simulink model "PubIfDecisionLM_MDL"  (R2020b)
settings: configuration reference "DspaceConfig" (kept outside this file)
PostLoadFcn:
  | if any(exist('dsrtsu_mdlpostloadfcn', 'file') ~= 0), dsrtsu_mdlpostloadfcn('Execute', bdroot); end
InitFcn:
  | , if any(exist('dsmpb_private', 'file') ~= 0), dsmpb_private('dsmpb_mdlclblib', 'Init', bdroot); end,
undefined symbols (not defined in the file or in its folder): OFM_OBJ_FUSIONTYPE_E, OFM_OBJ_MOVINGSTATE_E, OFM_OBJ_ORIENTATION_E, OFM_OBJ_TYPE_E, P_LM_Cyc, P_LM_EMLHistKapRcdBufSize, P_LM_EMLHistTrajBaseDis, P_LM_EMLHistTrajPNum, P_LM_EMLKapCorrMaxThre, P_LM_EMLMinKapThre, P_LM_EMLPathDisDiffThre, P_LM_EMLQuaFiltPar, P_LM_EMLTurnActKapThre, P_LM_EMLValidQuaThre, P_LM_FntPath1Disgap, P_LM_FntPath1MinDis, P_LM_FntPath1Timegap, P_LM_FntPath2Disgap, P_LM_FntPath2MinDis, P_LM_FntPath2Timegap, P_LM_FntPath3Disgap, P_LM_FntPath3MinDis, P_LM_FntPath3Timegap, P_LM_FusBLParFiltP, P_LM_FusEVDifC2Thre, P_LM_FusEVOPath1AllVSLDisThre, P_LM_FusEVOPath1AllVSLLostNumThre, P_LM_FusEVOPath1AllVSLQuaThre, P_LM_FusEVOPath1OTLFacNLC, P_LM_FusOTLQuaThre, P_LM_FusOTLSW, P_LM_FusParC0Index, P_LM_FusParC1Index, P_LM_FusParC2Index, P_LM_FusParC3Index, P_LM_FusVSLQuaThre, P_LM_FusVSLSW, P_LM_FusVSLValidSteerWheerAngThre, P_LM_FusVSLValidVxvThre, P_LM_LaneWidth, P_LM_OTLBufTPInfoEvaFactor, P_LM_OTLObjNum, P_LM_OTLObjSelectAgeThre, P_LM_OTLObjSelectDxAssessVx, P_LM_OTLObjSelectDxThre, P_LM_OTLObjSelectVxThre, P_LM_OTLObjSelectVyAssessDx, P_LM_OTLObjSelectVyThre, P_LM_OTLTrajPntBaseDis, P_LM_OTLTrajStdThre, P_LM_VSLAvailLineNum, P_LM_VSLBLSDiffThre, P_LM_VSLBLSDisRatio, P_LM_VSLFusBLParFiltP_C1, P_LM_VSLFusBLParFiltP_C2, P_LM_VSLFusBLParFiltP_C3, P_LM_VSLFusBLParFiltP_Quality, P_LM_VSLHistTrajBaseDis, P_LM_VSLHistTrajPNum, P_LM_VSLLCC0diff ... (+18)
libraries: simulink x145, LM_LIB x43
(part 24 of 24)

== matlab function PubIfDecisionLM_MDL/Subsystem2/LM_EML/LM_EMLRearPath1/MATLAB Function ==
  data: LM_EMLHistTrajVectX input; LM_EMLRearPath1P output; LM_EMLHistTrajVectY input; LM_EMLHistPEndPos input; LM_EMLHistPFristPos input; LM_EMLHistPNum input; LM_RearPath1Dis input; LM_RearPath2Dis input; LM_RearPath3Dis input; LM_EMLRearPath1Qulity output; LM_EMLRearPath2P output; LM_EMLRearPath2Qulity output; LM_EMLRearPath3P output; LM_EMLRearPath3Qulity output
function [LM_EMLRearPath1P,LM_EMLRearPath1Qulity,LM_EMLRearPath2P,LM_EMLRearPath2Qulity,LM_EMLRearPath3P,LM_EMLRearPath3Qulity] = ...
    fcn(LM_EMLHistTrajVectX,LM_EMLHistTrajVectY,LM_EMLHistPEndPos,LM_EMLHistPFristPos,LM_EMLHistPNum,LM_RearPath1Dis,LM_RearPath2Dis,LM_RearPath3Dis)
% 初始化拟合用dx,dy buffer
P_LM_EMLHistPNum = 80;
t_index = uint8(zeros(1,P_LM_EMLHistPNum));
if LM_EMLHistPNum > P_LM_EMLHistPNum
    if LM_EMLHistPEndPos == 1
        t_index(1) = uint8(1);
        for i = 2:P_LM_EMLHistPNum
            t_index(i) = uint8(P_LM_EMLHistPNum+2-i);
        end
    elseif LM_EMLHistPEndPos == P_LM_EMLHistPNum
        for i = 1:P_LM_EMLHistPNum
            t_index(i) = uint8(P_LM_EMLHistPNum+1-i);
        end
    else
        for i = 1:P_LM_EMLHistPNum
            if i <= LM_EMLHistPEndPos
                t_index(i) = uint8(LM_EMLHistPEndPos+1-i);
            else
                t_index(i) = uint8(P_LM_EMLHistPNum+1-(i-LM_EMLHistPEndPos));
            end
        end
    end
else
    for i = 1:P_LM_EMLHistPNum
            if i <= LM_EMLHistPEndPos
                t_index(i) = uint8(LM_EMLHistPEndPos+1-i);
            else
                t_index(i) = 1;
            end
    end
end

%% 后方第一段轨迹拟合
P_LM_EMLHPFitBuffSize = 80;
t_hpx = single(zeros(P_LM_EMLHPFitBuffSize,1));
t_hpy = single(zeros(P_LM_EMLHPFitBuffSize,1));
t_pnum = uint8(0);
if LM_EMLHistPNum > P_LM_EMLHistPNum
    t_fornum = uint8(P_LM_EMLHistPNum);
else
    t_fornum = uint8(LM_EMLHistPNum);
end
for i = 1:t_fornum
    if abs(LM_EMLHistTrajVectX(t_index(i))) <= LM_RearPath1Dis
        t_pnum = t_pnum + 1;
        t_hpx(t_pnum) = LM_EMLHistTrajVectX(t_index(i));
        t_hpy(t_pnum) = LM_EMLHistTrajVectY(t_index(i));
    end
end
if t_pnum ~=0
    if t_pnum < P_LM_EMLHPFitBuffSize 
        for i = t_pnum+1:P_LM_EMLHPFitBuffSize
            t_hpx(i) = t_hpx(t_pnum);
            t_hpy(i) = t_hpy(t_pnum);
        end
    end
    
    % 第1段参数拟合
    LM_EMLRearPath1P = polyfit(t_hpx,t_hpy,3);
    % 第一段拟合误差计算
    t_fity = polyval(LM_EMLRearPath1P,t_hpx);
    t_sumerry = single(0);
    for i=1:t_pnum
        t_erry = single((t_hpy(i) - t_fity(i))^2);
        t_sumerry = t_sumerry + t_erry;
    end
    t_quality = interpolate(single(0.5),single(1),single(3),single(0),single(t_sumerry));
    %由轨迹点个数求轨迹质量影响因子，当轨迹点小于7个时，轨迹质量影响因子为0；当轨迹点大于17个时，轨迹质量影响因子为1
    t_factor = interpolate(single(7),single(0),single(17),single(1),single(t_pnum));
    %轨迹质量= 轨迹质量*轨迹质量影响因子
    LM_EMLRearPath1Qulity = single(t_quality * t_factor);
    LM_EMLRearPath1Qulity = min(LM_EMLRearPath1Qulity,0.95);
    
% 轨迹质量计算 考虑历史轨迹点长度，及拟合误差
%  LM_EMLRearPath1Qulity = single(0.9);
else 
    LM_EMLRearPath1P = single([0 0 0 0]);
    LM_EMLRearPath1Qulity = single(0);
end

%%
LM_EMLHistMaxDis = abs(LM_EMLHistTrajVectX(LM_EMLHistPFristPos));
%% 后方第二段轨迹拟合
if LM_EMLHistMaxDis > LM_RearPath1Dis + 10
    t_pnum = uint8(0);
    for i = 1:t_fornum
        if abs(LM_EMLHistTrajVectX(t_index(i))) > LM_RearPath1Dis && abs(LM_EMLHistTrajVectX(t_index(i))) <= LM_RearPath2Dis
            t_pnum = t_pnum + 1;
            t_hpx(t_pnum) = LM_EMLHistTrajVectX(t_index(i));
            t_hpy(t_pnum) = LM_EMLHistTrajVectY(t_index(i));
        end
    end
    if t_pnum < P_LM_EMLHPFitBuffSize && t_pnum ~= 0
%         t_hpx(t_pnum+1:end) = t_hpx(t_pnum);
%         t_hpy(t_pnum+1:end) = t_hpy(t_pnum);
        for i = t_pnum+1:P_LM_EMLHPFitBuffSize
            t_hpx(i) = t_hpx(t_pnum);
            t_hpy(i) = t_hpy(t_pnum);
        end
    end
    % 第2段参数拟合
    LM_EMLRearPath2P = polyfit(t_hpx,t_hpy,3);
    % 第2段拟合误差计算
    t_fity = polyval(LM_EMLRearPath2P,t_hpx);
    t_sumerry = single(0);
    for i=1:t_pnum
        t_erry = single((t_hpy(i) - t_fity(i))^2);
        t_sumerry = t_sumerry + t_erry;
    end
    %由拟合误差求轨迹quality，当拟合误差小于0.5时，轨迹质量为1；当拟合误差大于3时，轨迹质量为0，否则轨迹质量插值
    t_quality = interpolate(0.5,1,3,0,t_sumerry);
    %由轨迹点个数求轨迹质量影响因子，当轨迹点小于7个时，轨迹质量影响因子为0；当轨迹点大于17个时，轨迹质量影响因子为1
    t_factor = interpolate(7,0,17,1,t_pnum);
    %轨迹质量= 轨迹质量*轨迹质量影响因子
    LM_EMLRearPath2Qulity = single(t_quality * t_factor);
    LM_EMLRearPath2Qulity = min(LM_EMLRearPath2Qulity,0.95);
%     LM_EMLRearPath2Qulity = single(0.9);
    
else
    LM_EMLRearPath2P = single([0 0 0 0]);
    LM_EMLRearPath2Qulity = single(0);
end
%% 后方第3段轨迹拟合
if LM_EMLHistMaxDis > LM_RearPath2Dis + 10
    t_pnum = uint8(0);
    for i = 1:t_fornum
        if abs(LM_EMLHistTrajVectX(t_index(i))) > LM_RearPath2Dis && abs(LM_EMLHistTrajVectX(t_index(i))) <= LM_RearPath3Dis
            t_pnum = t_pnum + 1;
            t_hpx(t_pnum) = LM_EMLHistTrajVectX(t_index(i));
            t_hpy(t_pnum) = LM_EMLHistTrajVectY(t_index(i));
        end
    end
    if t_pnum < P_LM_EMLHPFitBuffSize && t_pnum ~= 0
%         t_hpx(t_pnum+1:end) = t_hpx(t_pnum);
%         t_hpy(t_pnum+1:end) = t_hpy(t_pnum);
        for i = t_pnum+1:P_LM_EMLHPFitBuffSize
            t_hpx(i) = t_hpx(t_pnum);
            t_hpy(i) = t_hpy(t_pnum);
        end
    end
    % 第3段参数拟合
    LM_EMLRearPath3P = polyfit(t_hpx,t_hpy,3);
    % 第3段拟合误差计算
    t_fity = polyval(LM_EMLRearPath3P,t_hpx);
    t_sumerry = single(0);
    for i=1:t_pnum
        t_erry = single((t_hpy(i) - t_fity(i))^2);
        t_sumerry = t_sumerry + t_erry;
    end
    %由拟合误差求轨迹quality，当拟合误差小于0.5时，轨迹质量为1；当拟合误差大于3时，轨迹质量为0，否则轨迹质量插值
    t_quality = interpolate(single(0.5),single(1),single(3),single(0),single(t_sumerry));
    %由轨迹点个数求轨迹质量影响因子，当轨迹点小于7个时，轨迹质量影响因子为0；当轨迹点大于17个时，轨迹质量影响因子为1
    t_factor = interpolate(single(7),single(0),single(17),single(1),single(t_pnum));
    %轨迹质量= 轨迹质量*轨迹质量影响因子
    LM_EMLRearPath3Qulity = single(t_quality * t_factor);
    LM_EMLRearPath3Qulity = min(LM_EMLRearPath3Qulity,0.95);
%     LM_EMLRearPath3Qulity = single(0.9);
    
else
    LM_EMLRearPath3P = single([0 0 0 0]);
    LM_EMLRearPath3Qulity = single(0);
end
end
function out = interpolate(x1,z1,x2,z2,Raw)
if Raw<=x1
    out = single(z1);
else
    if Raw>=x2
        out = single(z2);
    else
        t_out = single((Raw-x1)*(z2-z1));
        t_out = single(t_out/(x2-x1));
        t_out = single(z1)+t_out;
        out = t_out;
    end
end
end

== matlab function PubIfDecisionLM_MDL/Subsystem2/LM_Fusion1/LM_FusBaseLineFilt/LM_FusBaseLineInfoFilt/LM_FusBLFntPath1InfoFilt/LM_FusBLPathQuliatyFilt/MATLAB Function ==
  data: u1 input; y output; yk1 input
function y = fcn(u1,yk1)
y = single(u1);
if isnan(u1)
    if isnan(yk1)
        y = single(0);
    else
        if yk1 ~= 0
            y = single(yk1);
        else
            y = single(0);
        end
    end
end

== matlab function PubIfDecisionLM_MDL/Subsystem2/LM_Fusion1/LM_FusBaseLineFilt/LM_FusBaseLineInfoFilt/LM_FusBLFntPath1InfoFilt/LM_Fus_BLFntPathC0Filt/MATLAB Function ==
  data: u1 input; y output; yk1 input
function y = fcn(u1,yk1)
y = single(u1);
if isnan(u1)
    if isnan(yk1)
        y = single(0);
    else
        if yk1 ~= 0
            y = single(yk1);
        else
            y = single(0);
        end
    end
end

== matlab function PubIfDecisionLM_MDL/Subsystem2/LM_Fusion1/LM_FusBaseLineFilt/LM_FusBaseLineInfoFilt/LM_FusBLFntPath1InfoFilt/LM_Fus_BLPath3C3Filt/MATLAB Function ==
  data: u1 input; y output; yk1 input
function y = fcn(u1,yk1)
y = single(u1);
if isnan(u1)
    if isnan(yk1)
        y = single(0);
    else
        if yk1 ~= 0
            y = single(yk1);
        else
            y = single(0);
        end
    end
end

== matlab function PubIfDecisionLM_MDL/Subsystem2/LM_Fusion1/LM_FusBaseLineFilt/LM_FusBaseLineInfoFilt/LM_FusBLFntPath1InfoFilt/LM_Fus_BLPathC1Filt/MATLAB Function ==
  data: u1 input; y output; yk1 input
function y = fcn(u1,yk1)
y = single(u1);
if isnan(u1)
    if isnan(yk1)
        y = single(0);
    else
        if yk1 ~= 0
            y = single(yk1);
        else
            y = single(0);
        end
    end
end

== matlab function PubIfDecisionLM_MDL/Subsystem2/LM_Fusion1/LM_FusBaseLineFilt/LM_FusBaseLineInfoFilt/LM_FusBLFntPath1InfoFilt/LM_Fus_BLPathC2Filt/MATLAB Function ==
  data: u1 input; y output; yk1 input
function y = fcn(u1,yk1)
y = single(u1);
if isnan(u1)
    if isnan(yk1)
        y = single(0);
    else
        if yk1 ~= 0
            y = single(yk1);
        else
            y = single(0);
        end
    end
end

== matlab function PubIfDecisionLM_MDL/Subsystem2/LM_Fusion1/LM_FusRatioCalc/LM_Fusion_EV/LM_FusEMLAndVSLRatioCalc/LM_Fusion_FntPathK/LM_Fusion_VSL_EMLPath1KCalc1 ==
  data: LM_VSLFntPath1Quality input; LM_VSLFntPath2Quality input; LM_VSLFntPath3Quality input; LM_FusEVFntPath1VSLK output; LM_FusEVFntPath2VSLK output; LM_FusEVFntPath3VSLK output; LM_EMLFntPath1Quality input; LM_EMLFntPath2Quality input; LM_EMLFntPath3Quality input; LM_FusEVdiffValid input; LM_FusEVFntPath1EMLK output; LM_FusEVFntPath2EMLK output; LM_FusEVFntPath3EMLK output; LM_ComLineLostNum input; LM_VSLBaseDis input; DIR_TurnLeftValid input; DIR_TurnRightValid input; DIR_LC2LeValid input; DIR_LC2RigValid input; vxvRefMs input
 function [LM_FusEVFntPath1VSLK,LM_FusEVFntPath2VSLK,LM_FusEVFntPath3VSLK,LM_FusEVFntPath1EMLK,LM_FusEVFntPath2EMLK,LM_FusEVFntPath3EMLK] = fcn(LM_VSLFntPath1Quality,LM_VSLFntPath2Quality,LM_VSLFntPath3Quality,...
    LM_EMLFntPath1Quality,LM_EMLFntPath2Quality,LM_EMLFntPath3Quality,LM_FusEVdiffValid,LM_ComLineLostNum,LM_VSLBaseDis, DIR_TurnLeftValid, DIR_TurnRightValid, DIR_LC2LeValid, DIR_LC2RigValid, vxvRefMs)

%% Parameter Configuration

t_flg = uint8(0); % 0 fus ; 1 VSL ; 2 EML
t_FusFntPath1VSLK = single(0);
t_FusFntPath2VSLK = single(0);
t_FusFntPath3VSLK = single(0);

t_FusFntPath1EMLK = single(1);
t_FusFntPath2EMLK = single(1);
t_FusFntPath3EMLK = single(1);


% 如果车辆掉头，轨迹完全用EML
if DIR_TurnLeftValid == true || DIR_TurnRightValid == true || (DIR_LC2LeValid ~= true && DIR_LC2RigValid ~= true && LM_FusEVdiffValid == true)    
    t_flg = uint8(2);
else
%% VSL 三段轨迹
    if LM_VSLFntPath3Quality ~= 0 
        if LM_VSLFntPath1Quality >= 0.3  %三段轨迹且车道线质量较高，清晰,道路模型输出VSL模型
            t_flg = uint8(1);
        elseif LM_VSLFntPath1Quality >= 0.1    %三段轨迹且车道线质量较差,如果丢失少于两条车道线则输出VSL否则输出EML
            if LM_ComLineLostNum <= 2
                t_flg = uint8(1);
            else
                t_flg = uint8(2);
            end
        else
            t_flg = uint8(2);  % 摄像头车道线质量太低输出EML
        end
%VSL 两段轨迹
    elseif LM_VSLFntPath2Quality ~= 0 
        if LM_VSLFntPath1Quality >= 0.6 || (LM_VSLFntPath1Quality >= 0.3 && LM_ComLineLostNum <=2)          %VSL两段轨迹且车道线质量较高，清晰
            t_flg = uint8(1);
        elseif LM_VSLFntPath1Quality >= 0.1 && LM_ComLineLostNum <=2  % VSL两段轨迹，车道线质量较差，丢失车道线少于2条
            if DIR_LC2LeValid == true || DIR_LC2RigValid == true  %换道完全用VSL
                t_flg = uint8(1);
            else  % 车道保持，EML&VSL 融合
                % path1
                t_EMLQualtiyAdju = LM_EMLFntPath1Quality * 0.95;
                t_qualitysum = t_EMLQualtiyAdju + LM_VSLFntPath1Quality;
                t_FusFntPath1VSLK = LM_VSLFntPath1Quality/t_qualitysum;
                t_FusFntPath1EMLK = t_EMLQualtiyAdju/t_qualitysum;
                % path2
                t_EMLQualtiyAdju = LM_EMLFntPath2Quality * 0.75;
                t_qualitysum = t_EMLQualtiyAdju + LM_VSLFntPath2Quality;
                t_FusFntPath2VSLK = LM_VSLFntPath2Quality/t_qualitysum;
                t_FusFntPath2EMLK = t_EMLQualtiyAdju/t_qualitysum;
                % path3
                t_EMLQualtiyAdju = LM_EMLFntPath3Quality * 0.6;
                t_qualitysum = t_EMLQualtiyAdju + LM_VSLFntPath3Quality;
                t_FusFntPath3VSLK = LM_VSLFntPath3Quality/t_qualitysum;
                t_FusFntPath3EMLK = t_EMLQualtiyAdju/t_qualitysum;
            end
        else
            t_flg = uint8(2);
        end
    elseif LM_VSLFntPath1Quality ~= 0
        % EML三段轨迹
        if LM_VSLFntPath1Quality < 0.1 || LM_VSLBaseDis < 10
            t_flg = uint8(2);
        else
            if LM_EMLFntPath3Quality ~=0  %车速较快，
                t_flg = uint8(2);
            else
                if LM_EMLFntPath2Quality ~= 0 % EML存在第二段轨迹
                    if DIR_LC2LeValid == true || DIR_LC2RigValid == true  %换道完全用VSL
                        t_flg = uint8(1);
                    else
                        % path1
                        t_VSLQualtiyAdju = LM_VSLFntPath1Quality * 0.5;
                        t_qualitysum = t_VSLQualtiyAdju + LM_EMLFntPath1Quality;
                        t_FusFntPath1VSLK = t_VSLQualtiyAdju/t_qualitysum;
                        t_FusFntPath1EMLK = LM_EMLFntPath1Quality/t_qualitysum;
                        t_FusFntPath2VSLK = t_FusFntPath1VSLK;
                        t_FusFntPath2EMLK = t_FusFntPath1EMLK;
                        t_FusFntPath3VSLK = t_FusFntPath1VSLK;
                        t_FusFntPath3EMLK = t_FusFntPath1EMLK;  
                    end
                else % EML不存在第二段轨迹
                    if DIR_LC2LeValid == true || DIR_LC2RigValid == true   %换道完全用VSL
                        t_flg = uint8(1);
                    else  % 车道保持，EML&VSL 融合
                        % path1
                        t_EMLQualtiyAdju = LM_EMLFntPath1Quality * 0.95;
                        t_qualitysum = t_EMLQualtiyAdju + LM_VSLFntPath1Quality;
                        t_FusFntPath1VSLK = LM_VSLFntPath1Quality/t_qualitysum;
                        t_FusFntPath1EMLK = t_EMLQualtiyAdju/t_qualitysum;
                        % path2
                        t_FusFntPath2VSLK = t_FusFntPath1VSLK;
                        t_FusFntPath2EMLK = t_FusFntPath1EMLK;
                        t_FusFntPath3VSLK = t_FusFntPath1VSLK;
                        t_FusFntPath3EMLK = t_FusFntPath1EMLK;
                    end
                end
            end
        end
    end
end
if t_flg == 1
    LM_FusEVFntPath1EMLK = single(0);
    LM_FusEVFntPath2EMLK = single(0);
    LM_FusEVFntPath3EMLK = single(0);
    
    LM_FusEVFntPath1VSLK = single(1);
    if LM_VSLFntPath2Quality ~= 0
        LM_FusEVFntPath2VSLK = single(1);
    else
        LM_FusEVFntPath2VSLK = single(0);
        if LM_EMLFntPath2Quality ~= 0
            LM_FusEVFntPath2EMLK = single(1);
        end
    end
    if LM_VSLFntPath3Quality ~= 0
        LM_FusEVFntPath3VSLK = single(1);
    else
        LM_FusEVFntPath3VSLK = single(0);
        if LM_EMLFntPath3Quality ~= 0
            LM_FusEVFntPath3EMLK = single(1);
        end
    end
    
elseif t_flg ==2
    LM_FusEVFntPath1VSLK = single(0);
    LM_FusEVFntPath2VSLK = single(0);
    LM_FusEVFntPath3VSLK = single(0);
    LM_FusEVFntPath1EMLK = single(1);
    LM_FusEVFntPath2EMLK = single(1);
    LM_FusEVFntPath3EMLK = single(1);   
else
    LM_FusEVFntPath1VSLK = single(t_FusFntPath1VSLK);
    LM_FusEVFntPath2VSLK = single(t_FusFntPath2VSLK);
    LM_FusEVFntPath3VSLK = single(t_FusFntPath3VSLK);
    LM_FusEVFntPath1EMLK = single(t_FusFntPath1EMLK);
    LM_FusEVFntPath2EMLK = single(t_FusFntPath2EMLK);
    LM_FusEVFntPath3EMLK = single(t_FusFntPath3EMLK); 
end

%EML PATH1K Adjust
if ~(DIR_TurnLeftValid == true || DIR_TurnRightValid == true || DIR_LC2LeValid == true || DIR_LC2RigValid == true)
    if LM_ComLineLostNum <= 1
        if vxvRefMs >= 10
            LM_FusEVFntPath1EMLK = max(LM_FusEVFntPath1EMLK,single(0.6));
            LM_FusEVFntPath1VSLK = (single(1) - LM_FusEVFntPath1EMLK);
        elseif vxvRefMs >= 6 
            LM_FusEVFntPath1EMLK = max(LM_FusEVFntPath1EMLK,single(0.45));
            LM_FusEVFntPath1VSLK = (single(1) - LM_FusEVFntPath1EMLK);
        end
    end
    %EML PATH2&3K Adjust
    if LM_EMLFntPath2Quality >= single(0.55)
        LM_FusEVFntPath2EMLK = max(LM_FusEVFntPath2EMLK,single(0.5));
        LM_FusEVFntPath2VSLK = (single(1) - LM_FusEVFntPath2EMLK);
    end
    if LM_EMLFntPath3Quality >= single(0.45)
        LM_FusEVFntPath3EMLK = max(LM_FusEVFntPath3EMLK,single(0.4));
        LM_FusEVFntPath3VSLK = (single(1) - LM_FusEVFntPath3EMLK);
    end       
end

== stateflow chart PubIfDecisionLM_MDL/Subsystem2/LM_SigPrePro1/Subsystem1/LM_RFMLineInfoFilter/Chart10 ==
  state Lost
    en:LM_LINE_Filt = RFM_LINE;
    du:LM_LINE_Filt = RFM_LINE;
    ex:LM_LINE_Filt = RFM_LINE;
  state Exist
    en: LM_LINE_Filt = RFM_LINE；
    du:
    if LM_LINE_K1.dC0V == nan || LM_LINE_K1.dC1V == nan
    LM_LINE_Filt = RFM_LINE;
    else
    LM_LINE_Filt = RFM_LINE;
    LM_LINE_Filt.dC0V=LM_LINE_K1.dC0V+0.15*(RFM_LINE.dC0V-LM_LINE_K1.dC0V);
    LM_LINE_Filt.dC1V=LM_LINE_K1.dC1V+0.15*(RFM_LINE.dC1V-LM_LINE_K1.dC1V);
    LM_LINE_Filt.dC2V=LM_LINE_K1.dC2V+0.15*(RFM_LINE.dC2V-LM_LINE_K1.dC2V);
    LM_LINE_Filt.dC3V=LM_LINE_K1.dC3V+0.15*(RFM_LINE.dC3V-LM_LINE_K1.dC3V);
    LM_LINE_Filt.dDisFront=LM_LINE_K1.dDisFront+0.15*(RFM_LINE.dDisFront-LM_LINE_K1.dDisFront);
    end
  (default) -> Lost
  Lost -> Exist : [RFM_LINE.bIsLineExist==2]
  Exist -> Lost : [RFM_LINE.bIsLineExist==1]
  data: RFM_LINE input Bus: RFM_LINE_BUS; LM_LINE_Filt output Bus: RFM_LINE_BUS size=1 =0; LM_LINE_K1 input Bus: RFM_LINE_BUS

== stateflow chart PubIfDecisionLM_MDL/Subsystem2/LM_SigPrePro1/Subsystem1/LM_RFMLineInfoFilter/Chart11 ==
  state Lost
    en:LM_LINE_Filt = RFM_LINE;
    du:LM_LINE_Filt = RFM_LINE;
    ex:LM_LINE_Filt = RFM_LINE;
  state Exist
    en: LM_LINE_Filt = RFM_LINE；
    du:LM_LINE_Filt = RFM_LINE；
    LM_LINE_Filt.dC0V=LM_LINE_K1.dC0V+0.15*(RFM_LINE.dC0V-LM_LINE_K1.dC0V);
    LM_LINE_Filt.dC1V=LM_LINE_K1.dC1V+0.15*(RFM_LINE.dC1V-LM_LINE_K1.dC1V);
    LM_LINE_Filt.dC2V=LM_LINE_K1.dC2V+0.15*(RFM_LINE.dC2V-LM_LINE_K1.dC2V);
    LM_LINE_Filt.dC3V=LM_LINE_K1.dC3V+0.15*(RFM_LINE.dC3V-LM_LINE_K1.dC3V);
    LM_LINE_Filt.dDisFront=LM_LINE_K1.dDisFront+0.15*(RFM_LINE.dDisFront-LM_LINE_K1.dDisFront);
  (default) -> Lost
  Lost -> Exist : [RFM_LINE.bIsLineExist==2]
  Exist -> Lost : [RFM_LINE.bIsLineExist==1]
  data: RFM_LINE input Bus: RFM_LINE_BUS; LM_LINE_Filt output Bus: RFM_LINE_BUS size=1 =0; LM_LINE_K1 input Bus: RFM_LINE_BUS

== stateflow chart PubIfDecisionLM_MDL/Subsystem2/LM_VSL/LM_VSLFntPath/LM_VSLC0Calc1 ==
  state [LLC0,LRC0,RLC0,RRC0] = fcn1(t_LM_VSLLineExistVect,t_LM_VSLLineC0Vect,t_LM_VSLLineQualityVect,t_P_LM_LaneWidth) [function]
    (default) -> (junction 53)
    (junction 53) -> (junction 288) [order 1] : [t_LM_VSLLineExistVect(3)==2&&...
        | t_LM_VSLLineQualityVect(3)>=0.1]
    (junction 288) -> (junction 54) [order 1] : [~(t_LM_VSLLineC0Vect(2)-t_LM_VSLLineC0Vect(3)>=0.7*t_P_LM_LaneWidth&&...
        | t_LM_VSLLineC0Vect(2)-t_LM_VSLLineC0Vect(3)<=1.2*t_P_LM_LaneWidth)]
    (junction 54) -> (junction 319) [order 1] : [LM_VSLLineQualityVect(2)<LM_VSLLineQualityVect(3)]
    (junction 53) -> (junction 55) [order 2] : {%R1 not exist
        | LRC0=t_LM_VSLLineC0Vect(2);
        | RLC0=LRC0-t_P_LM_LaneWidth}
    (junction 288) -> (junction 291) [order 2] : {%R1 exist & Distance satisfied
        | LRC0=t_LM_VSLLineC0Vect(2);
        | RLC0=t_LM_VSLLineC0Vect(3)}
    (junction 54) -> (junction 321) [order 2] : {%L1 quality high
        | LRC0=t_LM_VSLLineC0Vect(2);
        | RLC0=LRC0-t_P_LM_LaneWidth}
    (junction 319) -> (junction 323) : {%R1 quality high
        | RLC0=t_LM_VSLLineC0Vect(3);
        | LRC0=RLC0+t_P_LM_LaneWidth}
    (junction 291) -> (junction 55)
    (junction 321) -> (junction 291)
    (junction 323) -> (junction 321)
    (junction 55) -> (junction 59)
    (junction 59) -> (junction 295) [order 1] : [t_LM_VSLLineExistVect(1)==2&&...
        | t_LM_VSLLineQualityVect(1)>=0.1]
    (junction 295) -> (junction 302) [order 1] : [~(t_LM_VSLLineC0Vect(1)-LRC0>=0.8*t_P_LM_LaneWidth&&...
        | t_LM_VSLLineC0Vect(1)-LRC0<=1.2*t_P_LM_LaneWidth)]
    (junction 59) -> (junction 297) [order 2] : {%L2 not exist
        | LLC0=LRC0+t_P_LM_LaneWidth}
    (junction 295) -> (junction 299) [order 2] : {%L2 exist & Distance satisfied
        | LLC0=t_LM_VSLLineC0Vect(1)}
    (junction 302) -> (junction 304) : {%L2 exist & Distance not satisfied
        | LLC0=LRC0+t_P_LM_LaneWidth}
    (junction 299) -> (junction 297)
    (junction 304) -> (junction 299)
    (junction 297) -> (junction 69)
    (junction 307) -> (junction 309) [order 1] : [~(RLC0-t_LM_VSLLineC0Vect(4)>=0.8*t_P_LM_LaneWidth&&...
        | RLC0-t_LM_VSLLineC0Vect(4)<=1.2*t_P_LM_LaneWidth)]
    (junction 69) -> (junction 307) [order 1] : [t_LM_VSLLineExistVect(4)==2&&...
        | t_LM_VSLLineQualityVect(4)>=0.1]
    (junction 69) -> (junction 74) [order 2] : {%R2 not exist
        | RRC0=RLC0-t_P_LM_LaneWidth}
    (junction 307) -> (junction 311) [order 2] : {%R2 exist & Distance satisfied
        | RRC0=t_LM_VSLLineC0Vect(4)}
    (junction 309) -> (junction 314) : {%R2 exist & Distance not satisfied
        | RRC0=RLC0-t_P_LM_LaneWidth}
    (junction 311) -> (junction 74)
    (junction 314) -> (junction 311)
    (junction 74) -> (junction 317)
  state [LLC0,LRC0,RLC0,RRC0] = fcn2(t_LM_VSLLineExistVect,t_LM_VSLLineC0Vect,t_LM_VSLLineQualityVect,t_P_LM_LaneWidth) [function]
    (default) -> (junction 112)
    (junction 112) -> (junction 114) : {RLC0=t_LM_VSLLineC0Vect(3);
        | LRC0=RLC0+t_P_LM_LaneWidth}
    (junction 114) -> (junction 376) [order 1] : [t_LM_VSLLineExistVect(1)==2&&...
        | t_LM_VSLLineQualityVect(1)>=0.1]
    (junction 376) -> (junction 356) [order 1] : [~(t_LM_VSLLineC0Vect(1)-LRC0>=0.8*t_P_LM_LaneWidth&&...
        | t_LM_VSLLineC0Vect(1)-LRC0<=1.2*t_P_LM_LaneWidth)]
    (junction 356) -> (junction 379) : {%L2exist & Distance not satisfied
        | LLC0=LRC0+t_P_LM_LaneWidth;}
    (junction 114) -> (junction 380) [order 2] : {%L2 not exist
        | LLC0=LRC0+t_P_LM_LaneWidth}
    (junction 376) -> (junction 378) [order 2] : {%L2exist & Distance satisfied
        | LLC0=t_LM_VSLLineC0Vect(1);}
    (junction 378) -> (junction 380)
    (junction 379) -> (junction 378)
    (junction 380) -> (junction 118)
    (junction 118) -> (junction 358) [order 1] : [t_LM_VSLLineExistVect(4)==2&&...
        | t_LM_VSLLineQualityVect(4)>=0.1]
    (junction 358) -> (junction 363) [order 1] : [~(RLC0-t_LM_VSLLineC0Vect(4)>=0.8*t_P_LM_LaneWidth&&...
        | RLC0-t_LM_VSLLineC0Vect(4)<=1.2*t_P_LM_LaneWidth)]
    (junction 118) -> (junction 128) [order 2] : {%R2 not exist
        | RRC0=RLC0-t_P_LM_LaneWidth}
    (junction 358) -> (junction 360) [order 2] : {%R2exist & Distance satisfied
        | RRC0=t_LM_VSLLineC0Vect(4);}
    (junction 363) -> (junction 365) : {%R2exist & Distance not satisfied
        | RRC0=RLC0-t_P_LM_LaneWidth;}
    (junction 360) -> (junction 128)
    (junction 365) -> (junction 360)
    (junction 128) -> (junction 133)
  state [LLC0,LRC0,RLC0,RRC0] = fcn3(t_LM_VSLLineExistVect,t_LM_VSLLineC0Vect,t_LM_VSLLineQualityVect,t_P_LM_LaneWidth) [function]
    (default) -> (junction 171)
    (junction 342) -> (junction 343) [order 1] : [t_LM_VSLLineC0Vect(1)-t_LM_VSLLineC0Vect(4)>=2.6*t_P_LM_LaneWidth&&...
        | t_LM_VSLLineC0Vect(1)-t_LM_VSLLineC0Vect(4)<=3.4*t_P_LM_LaneWidth]
    (junction 171) -> (junction 342) [order 1] : [t_LM_VSLLineExistVect(4)==2&&t_LM_VSLLineQualityVect(4)>=0.1]
    (junction 343) -> (junction 348) : {%L2,R2存在 & L2R2间距合理
        | LLC0=t_LM_VSLLineC0Vect(1);
        | LRC0=LLC0-(t_LM_VSLLineC0Vect(1)-t_LM_VSLLineC0Vect(4))/single(3);
        | RLC0=LRC0-(t_LM_VSLLineC0Vect(1)-t_LM_VSLLineC0Vect(4))/single(3);
        | RRC0=t_LM_VSLLineC0Vect(4);}
    (junction 171) -> (junction 335) [order 2]
    (junction 342) -> (junction 345) [order 2] : {%R2存在 & L2R2距离过大
        | LLC0=1.5*t_P_LM_LaneWidth;
        | LRC0=0.5*t_P_LM_LaneWidth;
        | RLC0=-0.5*t_P_LM_LaneWidth;
        | RRC0=-1.5*t_P_LM_LaneWidth;}
    (junction 335) -> (junction 337) [order 1] : [abs(t_LM_VSLLineC0Vect(1))>=2.1*t_P_LM_LaneWidth||...
        | abs(t_LM_VSLLineC0Vect(1))<=0.9*t_P_LM_LaneWidth]
    (junction 335) -> (junction 192) [order 2] : {%R2不存在 & L2C0合适
        | LLC0=t_LM_VSLLineC0Vect(1);
        | LRC0=LLC0-t_P_LM_LaneWidth;
        | RLC0=LRC0-t_P_LM_LaneWidth;
        | RRC0=RLC0-t_P_LM_LaneWidth;}
    (junction 337) -> (junction 339) : {%R2不存在 & L2C0过大或过小
        | LLC0=1.5*t_P_LM_LaneWidth;
        | LRC0=0.5*t_P_LM_LaneWidth;
        | RLC0=-0.5*t_P_LM_LaneWidth;
        | RRC0=-1.5*t_P_LM_LaneWidth;}
    (junction 339) -> (junction 192)
    (junction 345) -> (junction 339)
    (junction 348) -> (junction 345) [commented out]
    (junction 192) -> (junction 328)
  state [LLC0,LRC0,RLC0,RRC0] = fcn4(t_LM_VSLLineExistVect,t_LM_VSLLineC0Vect,t_LM_VSLLineQualityVect,t_P_LM_LaneWidth) [function]
    (default) -> (junction 230)
    (junction 230) -> (junction 330) [order 1] : [abs(t_LM_VSLLineC0Vect(4))>=2.1*t_P_LM_LaneWidth||...
        | abs(t_LM_VSLLineC0Vect(4))<=0.9*t_P_LM_LaneWidth]
    (junction 230) -> (junction 236) [order 2] : {%R2C0合适
        | RRC0=t_LM_VSLLineC0Vect(4);
        | RLC0=RRC0+t_P_LM_LaneWidth;
        | LRC0=RLC0+t_P_LM_LaneWidth;
        | LLC0=LRC0+t_P_LM_LaneWidth}
    (junction 330) -> (junction 332) : {%R2C0过大或过小
        | LLC0=1.5*t_P_LM_LaneWidth;
        | LRC0=0.5*t_P_LM_LaneWidth;
        | RLC0=-0.5*t_P_LM_LaneWidth;
        | RRC0=-1.5*t_P_LM_LaneWidth;}
    (junction 332) -> (junction 236)
    (junction 236) -> (junction 285)
  (default) -> (junction 4)
  (junction 4) -> (junction 6) [order 1] : [LM_VSLLineExistVect(2)==2&&LM_VSLLineQualityVect(2)>=0.1]
  (junction 4) -> (junction 8) [order 2]
  (junction 6) -> (junction 29) : {[LM_VSLLLC0,LM_VSLLRC0,LM_VSLRLC0,LM_VSLRRC0] = fcn1(LM_VSLLineExistVect,LM_VSLLineC0Vect,LM_VSLLineQualityVect,P_LM_LaneWidth)}
  (junction 8) -> (junction 10) [order 1] : [LM_VSLLineExistVect(3)==2&&LM_VSLLineQualityVect(3)>=0.1]
  (junction 8) -> (junction 12) [order 2]
  (junction 10) -> (junction 28) : {[LM_VSLLLC0,LM_VSLLRC0,LM_VSLRLC0,LM_VSLRRC0] = fcn2(LM_VSLLineExistVect,LM_VSLLineC0Vect,LM_VSLLineQualityVect,P_LM_LaneWidth)}
  (junction 12) -> (junction 15) [order 1] : [LM_VSLLineExistVect(1)==2&&LM_VSLLineQualityVect(1)>=0.1]
  (junction 12) -> (junction 17) [order 2]
  (junction 15) -> (junction 27) : {[LM_VSLLLC0,LM_VSLLRC0,LM_VSLRLC0,LM_VSLRRC0] = fcn3(LM_VSLLineExistVect,LM_VSLLineC0Vect,LM_VSLLineQualityVect,P_LM_LaneWidth)}
  (junction 17) -> (junction 20) [order 1] : [LM_VSLLineExistVect(4)==2&&LM_VSLLineQualityVect(4)>=0.1]
  (junction 17) -> (junction 24) [order 2] : {%所有车道线丢失
      | LM_VSLLLC0=1.5*P_LM_LaneWidth,LM_VSLLRC0=0.5*P_LM_LaneWidth;
      | LM_VSLRLC0=-0.5*P_LM_LaneWidth,LM_VSLRRC0=-1.5*P_LM_LaneWidth;}
  (junction 20) -> (junction 26) : {[LM_VSLLLC0,LM_VSLLRC0,LM_VSLRLC0,LM_VSLRRC0] = fcn4(LM_VSLLineExistVect,LM_VSLLineC0Vect,LM_VSLLineQualityVect,P_LM_LaneWidth)}
  (junction 26) -> (junction 24)
  (junction 27) -> (junction 26)
  (junction 28) -> (junction 27)
  (junction 29) -> (junction 28)
  (junction 24) -> (junction 38)
  data: LLC0 function_output single size=1; LRC0 function_output single size=1; RLC0 function_output single size=1; RRC0 function_output single size=1; t_LM_VSLLineExistVect function_input; t_LM_VSLLineC0Vect function_input; t_LM_VSLLineQualityVect function_input; t_P_LM_LaneWidth function_input; LLC0 function_output; LRC0 function_output; RLC0 function_output; RRC0 function_output; t_LM_VSLLineExistVect function_input; t_LM_VSLLineC0Vect function_input; t_LM_VSLLineQualityVect function_input; t_P_LM_LaneWidth function_input; LLC0 function_output single size=1; LRC0 function_output single size=1; RLC0 function_output single size=1; RRC0 function_output single size=1; t_LM_VSLLineExistVect function_input; t_LM_VSLLineC0Vect function_input; t_LM_VSLLineQualityVect function_input; t_P_LM_LaneWidth function_input; LLC0 function_output; LRC0 function_output; RLC0 function_output; RRC0 function_output; t_LM_VSLLineExistVect function_input; t_LM_VSLLineC0Vect function_input; t_LM_VSLLineQualityVect function_input; t_P_LM_LaneWidth function_input; LM_VSLLineC0Vect input; LM_VSLLineQualityVect input; LM_VSLLineExistVect input; LM_VSLLLC0 output single size=1; LM_VSLLRC0 output single size=1; LM_VSLRLC0 output single size=1; LM_VSLRRC0 output single size=1; P_LM_LaneWidth input

== matlab function PubIfDecisionLM_MDL/Subsystem2/LM_VSL/LM_VSLFntPath/LM_VSL_LineInfoEvalutaion/LM_VSL_LineInfoEvalutaion/LM_VSL_LineDiffEvalutaion/LM_VSL_BaseLineSelc ==
  data: LM_VSLLineQualityVect input; LM_VSLLineDisFntVect input; LM_VSLLineMaxDis input; LM_VSLLineMaxDisIndex input; LM_VSLLineMaxQuality input; LM_VSLLineMaxQualityIndex input; LM_VSLLineExistVect input; LM_VSLBLIndex output; LM_VSLBLFntDis output
function [LM_VSLBLIndex,LM_VSLBLFntDis] = fcn(LM_VSLLineQualityVect,LM_VSLLineDisFntVect,LM_VSLLineMaxDis,LM_VSLLineMaxDisIndex,LM_VSLLineMaxQuality,LM_VSLLineMaxQualityIndex,LM_VSLLineExistVect)
LM_VSLBLIndex = uint8(LM_VSLLineMaxQualityIndex);

P_LM_VSLL1Index = uint8(2);
P_LM_VSLR1Index = uint8(3);
t_flg = false;
%L1和R1均存在，且质量相等，选最长的为基准
if LM_VSLLineExistVect(P_LM_VSLL1Index) == 2 && LM_VSLLineExistVect(P_LM_VSLR1Index) == 2 && LM_VSLLineQualityVect(P_LM_VSLL1Index) == LM_VSLLineQualityVect(P_LM_VSLR1Index)
    if LM_VSLLineDisFntVect(P_LM_VSLL1Index) >= LM_VSLLineDisFntVect(P_LM_VSLR1Index)
        LM_VSLBLIndex = P_LM_VSLL1Index;
        t_flg = true;
    else
        LM_VSLBLIndex = P_LM_VSLR1Index;
        t_flg = true;
    end
end       
%L1存在
if LM_VSLLineExistVect(P_LM_VSLL1Index) == 2 && t_flg == false
    %L1质量最好，且有效长度最大
    if LM_VSLLineMaxDisIndex == P_LM_VSLL1Index && LM_VSLLineMaxQualityIndex == P_LM_VSLL1Index
        LM_VSLBLIndex = P_LM_VSLL1Index;
        t_flg = true;
    else
        if (LM_VSLLineQualityVect(P_LM_VSLL1Index) >= 0.6 || (LM_VSLLineMaxQuality - LM_VSLLineQualityVect(P_LM_VSLL1Index)) <= 0.2)...
                && (LM_VSLLineDisFntVect(P_LM_VSLL1Index) >= 30 || (LM_VSLLineMaxDis - LM_VSLLineDisFntVect(P_LM_VSLL1Index)) <= 15)
            LM_VSLBLIndex = P_LM_VSLL1Index;
            t_flg = true;
        end
    end 
end
if LM_VSLLineExistVect(P_LM_VSLR1Index) == 2 && t_flg == false
    if LM_VSLLineMaxDisIndex == P_LM_VSLR1Index && LM_VSLLineMaxQualityIndex == P_LM_VSLR1Index
        LM_VSLBLIndex = P_LM_VSLR1Index;
    else
        if (LM_VSLLineQualityVect(P_LM_VSLR1Index) >= 0.6 || (LM_VSLLineMaxQuality - LM_VSLLineQualityVect(P_LM_VSLR1Index)) <= 0.2)...
                && (LM_VSLLineDisFntVect(P_LM_VSLR1Index) >= 30 || (LM_VSLLineMaxDis - LM_VSLLineDisFntVect(P_LM_VSLR1Index)) <= 15)
            LM_VSLBLIndex = P_LM_VSLR1Index;
        end
    end
end
if LM_VSLBLIndex ~= uint8(0)
    LM_VSLBLFntDis = LM_VSLLineDisFntVect(LM_VSLBLIndex);
else
    LM_VSLBLFntDis = LM_VSLLineMaxDis;
end

== matlab function PubIfDecisionLM_MDL/Subsystem2/LM_VSL/LM_VSLFntPath/LM_VSL_LineInfoEvalutaion/LM_VSL_LineInfoEvalutaion/LM_VSL_LineDiffEvalutaion/LM_VSL_DiffMaxLineEvaluation3 ==
  data: LM_VSLBLIndex input; LM_VSLBLFntDis input; LM_VSLLineExistVect input; LM_VSLLineC0Vect input; LM_ComLineLostNum input; LM_VSLLineC1Vect input; LM_VSLLineC2Vect input; LM_VSLLineC3Vect input; LM_VSLDiffValid output; LM_VSLDiffValue output; Diffnum output; LM_VSLLineDisFntVect input; P_LM_VSLBLSDiffThre input; P_LM_VSLBLSDisRatio input
 function [LM_VSLDiffValid,LM_VSLDiffValue,Diffnum] = fcn(LM_VSLBLIndex,LM_VSLBLFntDis,LM_VSLLineExistVect,LM_VSLLineC0Vect,LM_ComLineLostNum,LM_VSLLineC1Vect,LM_VSLLineC2Vect,LM_VSLLineC3Vect,LM_VSLLineDisFntVect,P_LM_VSLBLSDiffThre,P_LM_VSLBLSDisRatio)

LM_VSLDiffValid = [false,false,false,false];
LM_VSLDiffValue = single((zeros(4,1)));
Distance = single(zeros(4,1));
Diffnum = single(0);
if LM_VSLBLFntDis <= 40
    t_disbase = 5;
elseif LM_VSLBLFntDis <= 80  && LM_VSLBLFntDis > 40
    t_disbase = 10;
elseif LM_VSLBLFntDis <= 120  && LM_VSLBLFntDis > 80
    t_disbase = 15;
else
    t_disbase = 15;
end
t_pnum = uint8(LM_VSLBLFntDis/t_disbase);
t_pnum = max(2,t_pnum);
if LM_ComLineLostNum <2
    for i=1:4
        if LM_VSLLineExistVect(i) == 2 && uint8(i) ~= LM_VSLBLIndex
            LM_VSLDiffValid(LM_VSLBLIndex)= true; 
            LM_VSLDiffValue(LM_VSLBLIndex) = single(0);
            Distance(LM_VSLBLIndex) = single(0);
            if LM_VSLLineDisFntVect(i) < single(40)
            Distance(i) = LM_VSLLineDisFntVect(LM_VSLBLIndex) - LM_VSLLineDisFntVect(i);
            else
             Distance(i) = single(0);
            end
            t_diffsum = single(0);
            dyn = single(zeros(11,1));
            dy  = single(zeros(11,1));
            for j = 1:t_pnum+1
                t_dx = single(j-1)*t_disbase;
                t_dyn = LM_VSLLineC0Vect(i) + LM_VSLLineC1Vect(i)*t_dx + LM_VSLLineC2Vect(i)*t_dx^2+LM_VSLLineC3Vect(i)*t_dx^3;
                t_dy = LM_VSLLineC0Vect(LM_VSLBLIndex) + LM_VSLLineC1Vect(LM_VSLBLIndex)*t_dx + LM_VSLLineC2Vect(LM_VSLBLIndex)*t_dx^2+LM_VSLLineC3Vect(LM_VSLBLIndex)*t_dx^3;
                dyn(j)= t_dyn;
                dy(j) = t_dy;
                t_diff = t_dyn - t_dy;
                t_diffsum = t_diffsum + t_diff;
            end
            t_diffmean = t_diffsum/single(t_pnum+1);
            t_diffisum = single(0);
           for k = 1:t_pnum+1
               t_diffi = (dyn(k) - t_diffmean - dy(k))^2;
               t_diffisum = t_diffisum + t_diffi;
           end
               t_variance = t_diffisum/single(t_pnum+1);
               LM_VSLDiffValue(i) = t_variance;
            if t_variance <=P_LM_VSLBLSDiffThre && Distance(i) <= P_LM_VSLBLSDisRatio * LM_VSLLineDisFntVect(i)
                LM_VSLDiffValid(i) = true;
            else
                LM_VSLDiffValid(i) = false;
            end
        end
    end
         
    for i=1:4
        if LM_VSLDiffValid(i) == true
            Diffnum = Diffnum +1;
        end
    end
end

== matlab function PubIfDecisionLM_MDL/Subsystem2/LM_VSL/LM_VSLFntPath/LM_VSL_LineInfoEvalutaion/LM_VSL_LineInfoEvalutaion/LM_VSL_LineDisEvaluation/If Action Subsystem1/LM_VSLLineMaxDisCalc ==
  data: LM_VSLLineMaxDis output; LM_VSLLineDisFntVect input; LM_VSLLineMaxDisIndex output; LM_VSLLineMeanDis output
 function [LM_VSLLineMaxDis,LM_VSLLineMaxDisIndex,LM_VSLLineMeanDis] = fcn(LM_VSLLineDisFntVect)
% LM_VSLLineDisSortIndexVect = uint8(zeros(4,1));
% 求最远距离及所在索引
[t_linemaxdis,t_linemaxdisindex] = max(LM_VSLLineDisFntVect);
% 判断最远距离车道线是否存在

    LM_VSLLineMaxDis = single(t_linemaxdis);
    LM_VSLLineMaxDisIndex = uint8(t_linemaxdisindex);   
    LM_VSLLineMeanDis = single(mean(LM_VSLLineDisFntVect));
  
%     [~,t_dissortindexvect] = sort(LM_VSLLineDisFntVect,'descend');
%     LM_VSLLineDisSortIndexVect = uint8(t_dissortindexvect);

== matlab function PubIfDecisionLM_MDL/Subsystem2/LM_VSL/LM_VSLFntPath/LM_VSL_LineInfoEvalutaion/LM_VSL_LineInfoEvalutaion/LM_VSL_LineQualityEvalutaion/If Action Subsystem1/LM_VSL_LineQualityEvaluation ==
  data: LM_VSLLineExistVect input; LM_VSLLineMaxQualiy output; LM_VSLLineMaxQualiyIndex output; LM_VSLLineMinQualiy output; LM_VSLLineMinQualiyIndex output; LM_VSLLineQualityVect input; LM_VSLLineMeanQuality output; LM_VSLLineQualityVar output
function [LM_VSLLineMaxQualiy,LM_VSLLineMaxQualiyIndex,LM_VSLLineMinQualiy,LM_VSLLineMinQualiyIndex,LM_VSLLineMeanQuality,LM_VSLLineQualityVar] = fcn(LM_VSLLineExistVect,LM_VSLLineQualityVect)

% find the line with max quailty
t_value = single(0);
t_index = uint8(0);
for i=1:4
    if LM_VSLLineQualityVect(i)>t_value
        t_value = LM_VSLLineQualityVect(i);
        t_index = uint8(i);
    end
end
% [t_linequality,t_linequalityindex] = max(LM_VSLLineQualityVect);
% LM_VSLLineMaxQualiy = single(t_linequality);
% LM_VSLLineMaxQualiyIndex = uint8(t_linequalityindex);
LM_VSLLineMaxQualiy = single(t_value);
LM_VSLLineMaxQualiyIndex = uint8(t_index);
% find the line with min quailty
% [t_linequality,t_linequalityindex] = min(LM_VSLLineQualityVect);
% LM_VSLLineMinQualiy = single(t_linequality);
% LM_VSLLineMinQualiyIndex = uint8(t_linequalityindex);

t_value = single(255);
t_index = uint8(0);
for i=1:4
    if LM_VSLLineQualityVect(i)<t_value
        t_value = LM_VSLLineQualityVect(i);
        t_index = uint8(i);
    end
end
LM_VSLLineMinQualiy = single(t_value);
LM_VSLLineMinQualiyIndex = uint8(t_index);        
% calculate mean value and varance for line quality
% LM_VSLLineMeanQuality = single(sum(LM_VSLLineQualityVect)/numel(find(LM_VSLLineQualityVect~=0)));
t_num=single(0);
for i=1:4
    if LM_VSLLineQualityVect(i)~=0
        t_num=t_num+1;
    end
end
LM_VSLLineMeanQuality = single(sum(LM_VSLLineQualityVect))/t_num;
    
t_varsum=single(0);
for i=1:4
    if LM_VSLLineExistVect(i) == 2 && LM_VSLLineQualityVect(i) ~=0
        t_var = (LM_VSLLineQualityVect(i) - LM_VSLLineMeanQuality)^2;
        t_varsum = t_varsum + t_var;
    end
end
LM_VSLLineQualityVar = t_varsum;

== stateflow chart PubIfDecisionLM_MDL/Subsystem2/LM_VSL/LM_VSLFntPath/LM_VSL_LineQualityCalc/LM_VSL_FntPath2QualityCalc/Chart ==
  state midstate2disappear
    en:
    t_times = uint8(0);
    temp = LM_VSLBaseDis/LM_FntPath2Dis;
    temp = min(single(1),temp);
    pathquality = temp * LM_VSLBaseQuality;
    du:
    t_times = t_times + uint8(1);
    temp = LM_VSLBaseDis/LM_FntPath2Dis;
    temp = min(single(1),temp);
    pathquality = temp * LM_VSLBaseQuality;
  state pathdisappear
    en:
    pathquality = single(0);
    du:
    pathquality = single(0);
    ex:
    pathquality = single(0);
  state midstate2appear
    en:
    t_times = uint8(0);
    pathquality = single(0);
    du:
    t_times = t_times + uint8(1);
    pathquality = single(0);
    ex:
    pathquality = single(0);
  state pathappear
    en:
    temp = LM_VSLBaseDis/LM_FntPath2Dis;
    temp = min(single(1),temp);
    pathquality = temp * LM_VSLBaseQuality;
    du:
    temp = LM_VSLBaseDis/LM_FntPath2Dis;
    temp = min(single(1),temp);
    pathquality = temp * LM_VSLBaseQuality;
  (default) -> pathdisappear
  midstate2disappear -> pathdisappear [order 1] : [~((LM_VSLBaseDis - LM_FntPath1Dis)>= (-P_LM_PathDisDiffThre)) ...
      | && t_times >= uint8(20)]
  pathdisappear -> midstate2appear : [(LM_VSLBaseDis - LM_FntPath1Dis)>= (-P_LM_PathDisDiffThre)]
  midstate2appear -> pathdisappear [order 1] : [~((LM_VSLBaseDis - LM_FntPath1Dis)>= (-P_LM_PathDisDiffThre))]
  pathappear -> midstate2disappear : [~((LM_VSLBaseDis - LM_FntPath1Dis)>= (-P_LM_PathDisDiffThre))]
  midstate2disappear -> pathappear [order 2] : [(LM_VSLBaseDis - LM_FntPath1Dis)>= (-P_LM_PathDisDiffThre)]
  midstate2appear -> pathappear [order 2] : [(LM_VSLBaseDis - LM_FntPath1Dis)>= (-P_LM_PathDisDiffThre) && t_times >= uint8(10)]
  data: LM_VSLBaseDis input; LM_FntPath2Dis input; pathquality output single size=1; LM_FntPath1Dis input; LM_VSLBaseQuality input; P_LM_PathDisDiffThre input; t_times local uint8 size=1; temp local single

== stateflow chart PubIfDecisionLM_MDL/Subsystem2/LM_VSL/LM_VSLFntPath/LM_VSL_LineQualityCalc/LM_VSL_FntPath3QualityCalc/Chart ==
  state midstate2disappear
    en:
    t_times = uint8(0);
    temp = LM_VSLBaseDis/LM_FntPath3Dis;
    temp = min(single(1),temp);
    pathquality = temp * LM_VSLBaseQuality;
    du:
    t_times = t_times + uint8(1);
    temp = LM_VSLBaseDis/LM_FntPath3Dis;
    temp = min(single(1),temp);
    pathquality = temp * LM_VSLBaseQuality;
  state pathdisappear
    en:
    pathquality = single(0);
    du:
    pathquality = single(0);
    ex:
    pathquality = single(0);
  state midstate2appear
    en:
    t_times = uint8(0);
    pathquality = single(0);
    du:
    t_times = t_times + uint8(1);
    pathquality = single(0);
    ex:
    pathquality = single(0);
  state pathappear
    en:
    temp = LM_VSLBaseDis/LM_FntPath3Dis;
    temp = min(single(1),temp);
    pathquality = temp * LM_VSLBaseQuality;
    du:
    temp = LM_VSLBaseDis/LM_FntPath3Dis;
    temp = min(single(1),temp);
    pathquality = temp * LM_VSLBaseQuality;
  (default) -> pathdisappear
  midstate2disappear -> pathdisappear [order 2] : [~((LM_VSLBaseDis - LM_FntPath2Dis)>= (-P_LM_PathDisDiffThre)) && t_times >= uint8(20)]
  pathdisappear -> midstate2appear : [(LM_VSLBaseDis - LM_FntPath2Dis)>= (-P_LM_PathDisDiffThre)]
  midstate2appear -> pathdisappear [order 1] : [~((LM_VSLBaseDis - LM_FntPath2Dis)>= (-P_LM_PathDisDiffThre))]
  pathappear -> midstate2disappear : [~((LM_VSLBaseDis - LM_FntPath2Dis)>= (-P_LM_PathDisDiffThre))]
  midstate2disappear -> pathappear [order 1] : [(LM_VSLBaseDis - LM_FntPath2Dis)>= (-P_LM_PathDisDiffThre)]
  midstate2appear -> pathappear [order 2] : [(LM_VSLBaseDis - LM_FntPath2Dis)>= (-P_LM_PathDisDiffThre) && t_times >= uint8(10)]
  data: LM_VSLBaseDis input; LM_FntPath2Dis input; pathquality output single size=1; LM_FntPath3Dis input; LM_VSLBaseQuality input; P_LM_PathDisDiffThre input; t_times local uint8 size=1; temp local single

== stateflow chart PubIfDecisionLM_MDL/Subsystem2/LM_VSL/LM_VSLFntPath/LM_VSL_LineQualityCalc/LM_VSL_FntPath3QualityCalc1/Chart ==
  state pathdisappear
    en:
    pathquality = single(0);
    du:
    pathquality = single(0);
    ex:
    pathquality = single(0);
  state midstate2disappear
    en:
    t_times = uint8(0);
    temp = LM_FntPath3Dis/LM_VSLBaseDis;
    temp = min(single(1),temp);
    pathquality = temp * LM_VSLBaseQuality;
    du:
    t_times = t_times + uint8(1);
    temp = LM_FntPath3Dis/LM_VSLBaseDis;
    temp = min(single(1),temp);
    pathquality = temp * LM_VSLBaseQuality;
  state midstate2appear
    en:
    t_times = uint8(0);
    pathquality = single(0);
    du:
    t_times = t_times + uint8(1);
    pathquality = single(0);
    ex:
    pathquality = single(0);
  state pathappear
    en:
    temp = LM_FntPath3Dis/LM_VSLBaseDis;
    temp = min(single(1),temp);
    pathquality = temp * LM_VSLBaseQuality;
    du:
    temp = LM_FntPath3Dis/LM_VSLBaseDis;
    temp = min(single(1),temp);
    pathquality = temp * LM_VSLBaseQuality;
  (default) -> pathdisappear
  midstate2disappear -> pathdisappear [order 2] : [~((LM_VSLBaseDis - LM_FntPath2Dis)>= (-P_LM_PathDisDiffThre)) && t_times >= uint8(20)]
  pathdisappear -> midstate2appear : [(LM_VSLBaseDis - LM_FntPath2Dis)>= (-P_LM_PathDisDiffThre)]
  midstate2appear -> pathdisappear [order 1] : [~((LM_VSLBaseDis - LM_FntPath2Dis)>= (-P_LM_PathDisDiffThre))]
  midstate2appear -> pathappear [order 2] : [(LM_VSLBaseDis - LM_FntPath2Dis)>= (-P_LM_PathDisDiffThre) && t_times >= uint8(10)]
  pathappear -> midstate2disappear : [~((LM_VSLBaseDis - LM_FntPath2Dis)>= (-P_LM_PathDisDiffThre))]
  midstate2disappear -> pathappear [order 1] : [(LM_VSLBaseDis - LM_FntPath2Dis)>= (-P_LM_PathDisDiffThre)]
  data: LM_VSLBaseDis input; LM_FntPath2Dis input; pathquality output single size=1; LM_FntPath3Dis input; LM_VSLBaseQuality input; P_LM_PathDisDiffThre input; t_times local uint8 size=1; temp local single

== stateflow chart PubIfDecisionLM_MDL/Subsystem2/LM_VSL/LM_VSLRearPath/LM_VSLC0Calc/LM_VSLC0Calc ==
  (default) -> (junction 1) : {LM_VSLLRC0=single(P_LM_LaneWidth*0.5)
      |  LM_VSLRLC0=single(-P_LM_LaneWidth*0.5)}
  (junction 1) -> (junction 7) [order 1] : [RFM_VSLLineblsLineExistVect(2)==1||RFM_VSLLineblsQualityVect(2)<0.1]
  (junction 7) -> (junction 21) [order 1] : [RFM_VSLLineblsLineExistVect(3)==1||RFM_VSLLineblsQualityVect(3)<0.1]
  (junction 21) -> (junction 23) [order 1] : [RFM_VSLLineblsLineExistVect(1)==1||RFM_VSLLineblsQualityVect(1)<0.1]
  (junction 23) -> (junction 31) [order 1] : [RFM_VSLLineblsLineExistVect(4)==1||RFM_VSLLineblsQualityVect(4)<0.1]
  (junction 1) -> (junction 51) [order 2]
  (junction 7) -> (junction 9) [order 2] : {%R1满足条件,L1不满足条件
      | LM_VSLLRC0=RFM_VSLLineC0Vect(3)+P_LM_LaneWidth
      | LM_VSLRLC0=RFM_VSLLineC0Vect(3)}
  (junction 21) -> (junction 28) [order 2]
  (junction 23) -> (junction 35) [order 2] : {%R2存在且车道线质量大于0.1,L2不满足条件
      | LM_VSLLRC0=RFM_VSLLineC0Vect(4)+2*P_LM_LaneWidth
      | LM_VSLRLC0=RFM_VSLLineC0Vect(4)+P_LM_LaneWidth}
  (junction 31) -> (junction 33)
  (junction 51) -> (junction 53) [order 1] : [RFM_VSLLineblsLineExistVect(3)==1||RFM_VSLLineblsQualityVect(3)<0.1]
  (junction 53) -> (junction 55) : {%L1满足条件,R1不满足条件
      | LM_VSLLRC0=RFM_VSLLineC0Vect(2)
      | LM_VSLRLC0=RFM_VSLLineC0Vect(2)-P_LM_LaneWidth}
  (junction 51) -> (junction 3) [order 2] : {%L1满足条件,R1满足条件
      | LM_VSLLRC0=RFM_VSLLineC0Vect(2)
      | LM_VSLRLC0=RFM_VSLLineC0Vect(3)}
  (junction 28) -> (junction 39) [order 1] : [RFM_VSLLineblsLineExistVect(4)==2&&RFM_VSLLineblsQualityVect(4)>=0.1]
  (junction 39) -> (junction 42) [order 1] : [RFM_VSLLineblsQualityVect(4)>RFM_VSLLineblsQualityVect(1)]
  (junction 28) -> (junction 25) [order 2] : {%L2满足条件,R2不满足条件
      | LM_VSLLRC0=RFM_VSLLineC0Vect(1)-P_LM_LaneWidth
      | LM_VSLRLC0=RFM_VSLLineC0Vect(1)-2*P_LM_LaneWidth}
  (junction 39) -> (junction 44) [order 2] : {%L2,R2满足条件,L2质量高
      | LM_VSLLRC0=RFM_VSLLineC0Vect(1)-P_LM_LaneWidth
      | LM_VSLRLC0=RFM_VSLLineC0Vect(1)-2*P_LM_LaneWidth}
  (junction 42) -> (junction 45) : {%L2,R2满足条件,R2质量高
      | LM_VSLLRC0=RFM_VSLLineC0Vect(4)+2*P_LM_LaneWidth
      | LM_VSLRLC0=RFM_VSLLineC0Vect(4)+P_LM_LaneWidth}
  (junction 9) -> (junction 55)
  (junction 55) -> (junction 3)
  (junction 25) -> (junction 9)
  (junction 44) -> (junction 25)
  (junction 45) -> (junction 44)
  (junction 35) -> (junction 45)
  (junction 33) -> (junction 35)
  (junction 3) -> (junction 5)
  data: RFM_VSLLineC0Vect input; RFM_VSLLineblsLineExistVect input; RFM_VSLLineblsQualityVect input; P_LM_LaneWidth input; LM_VSLLRC0 output; LM_VSLRLC0 output

== matlab function PubIfDecisionLM_MDL/Subsystem2/LM_VSL/LM_VSLRearPath/LM_VSLC0Calc/LM_VSLC0Check ==
  data: LM_VSLLRC0 input; LM_VSLRLC0 input; LM_VSLLRC0Adju output; LM_VSLRLC0Adju output; LM_VSLLineExistVect input; LM_VSLLineQualityVect input
function [LM_VSLLRC0Adju,LM_VSLRLC0Adju] = fcn(LM_VSLLRC0,LM_VSLRLC0,LM_VSLLineExistVect,LM_VSLLineQualityVect)
LM_VSLLRC0Adju = min(LM_VSLLRC0,3.75);
LM_VSLRLC0Adju = max(LM_VSLRLC0,-3.75);

%判断d(LRC0-RLC0)
P_LM_LaneWidth = single(3.5);
t_dis = LM_VSLLRC0Adju - LM_VSLRLC0Adju;
if ~(t_dis <= (P_LM_LaneWidth * single(1.2)) && t_dis >= (P_LM_LaneWidth * single(0.8)))
    
    %LR&RL均存在
    if LM_VSLLineExistVect(2) == 2 && LM_VSLLineExistVect(3) ==2
        
        %LR质量高
        if LM_VSLLineQualityVect(2) >0.1
            LM_VSLRLC0Adju = LM_VSLLRC0Adju - P_LM_LaneWidth;
        else
            LM_VSLLRC0Adju = LM_VSLRLC0Adju + P_LM_LaneWidth;
        end
        
        %LR存在,RL不存在
    elseif LM_VSLLineExistVect(2) == 2 && LM_VSLLineExistVect(3) ~=2
        LM_VSLRLC0Adju = LM_VSLLRC0Adju - P_LM_LaneWidth;
        
        %RL存在,LR不存在
    elseif LM_VSLLineExistVect(2) ~= 2 && LM_VSLLineExistVect(3) ==2
        LM_VSLLRC0Adju = LM_VSLRLC0Adju + P_LM_LaneWidth;
        
        
    end
end
end
